simulink model "SVM_CG"  (R2024a)
settings: Solver=FixedStepDiscrete  StartTime=0.0  StopTime=Inf  RelTol=1e-3  EnableMultiTasking=on
undefined symbols (not defined in the file): Down, GPTRIP1SEL, T_period, TZ1, Up, Vdc
libraries: c2802xlib x3, simulink x1
settings Model: ExtModeTrigDuration=8  Creator=kareem  LastModifiedBy=kareem
settings OptimizationCC: DefaultUnderspecifiedDataType=single  EnhancedBackFolding=on  PassReuseOutputArgsAs=Individual arguments  MaxStackSize=1024  OptimizeBlockOrder=speed  DifferentSizesBufferReuse=on  OptimizationCustomize=off  EfficientTunableParamExpr=on
settings DebuggingCC: ParameterTunabilityLossMsg=error
settings HardwareCC: ProdBitPerChar=16  ProdBitPerInt=16  ProdBitPerPointer=32  ProdBitPerSizeT=32  ProdBitPerPtrDiffT=32  ProdLargestAtomicInteger=Integer  ProdLargestAtomicFloat=None  ProdWordSize=16  ProdLongLongMode=on  ProdHWDeviceType=Texas Instruments->C2000  HardwareBoardFeatureSet=SoCBlockset
settings SFSimCC: MATLABDynamicMemAlloc=off
settings RTWCC: Description=Embedded Coder  SystemTargetFile=ert.tlc  HardwareBoard=TI Delfino F28379D LaunchPad  TemplateMakefile=ert_default_tmf  Toolchain=Texas Instruments Code Composer Studio (C2000)  CodeProfilingSaveOptions=MetricsOnly
settings CodeAppCC: ForceParamTrailComments=on  IgnoreCustomStorageClasses=off  OperatorAnnotations=on  SimulinkDataObjDesc=on  SFDataObjDesc=on  InsertBlockDesc=on
settings ERTTargetCC: CodeReplacementLibrary=TI C28x  SupportContinuousTime=on  ExtModeTransport=4  ExtModeStaticAlloc=on  ExtModeAutomaticAllocSize=off  ExtModeStaticAllocSize=10000  ExtModeMexFile=ext_xcp  ExtModeIntrfLevel=Level2 - Open

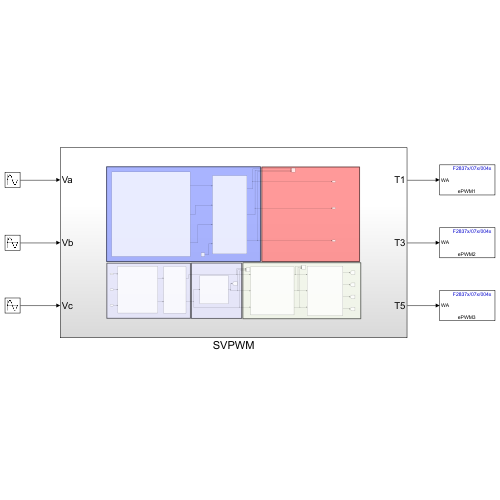
[thumbnail: Simulink's stored preview of the top-level diagram]
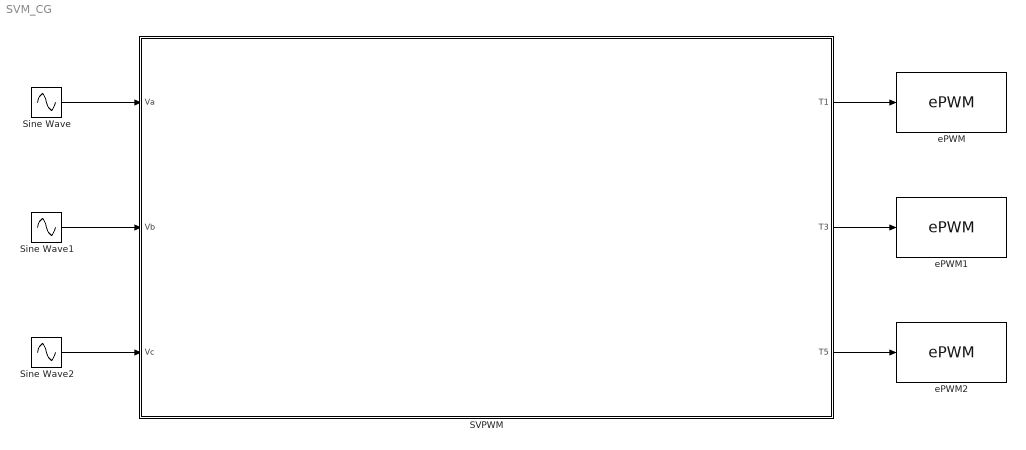
== system SVM_CG ==
  SVPWM : Subsystem
  Sine Wave : Sin  SampleTime=0
  Sine Wave1 : Sin  SampleTime=0
  Sine Wave2 : Sin  SampleTime=0
  ePWM : c2802xlib/ePWM  PwmType=C2000_Type4  useModule=ePWM1  ePWMxLINKTBPRD=Not Linked  periodUnits=Clock cycles  timerSource=Specify via dialog  timerPeriod_clk=10000  timerPeriod_sec=0.0001  tbshadow=Counter equals to zero  countingMode=Up-Down  phaseActiveEnable=Disable  phaseDirection=Count down after sync  phaseActive=0  synchronizationEnable=off  dcaevt1Sync=off  dcbevt1Sync=off  synchronizationOption=Disable  dcbevt1SyncOut=off  dcaevt1SyncOut=off  cmpdSyncOut=off  cmpcSyncOut=off  cmpbSyncOut=off  zeroSyncOut=off  swfSyncOut=off  perSynchronizationOption=Counter equals to period (CTR=PRD)  clockPrescale=1  HSclockPrescale=1  enswap=off  ePWMxAStatus=on  ePWMxAactionLogic1=Do nothing  ePWMxAactionLogic2=Do nothing  ePWMxAactionLogic3=Clear  ePWMxAactionLogic4=Set  ePWMxAactionLogic5=Do nothing  ePWMxAactionLogic6=Do nothing  ePWMxACSFenable=off  ePWMxACSFvalue=Forcing disable  ePWMxASFreload=Zero  ePWMxBStatus=on  ePWMxBactionLogic1=Do nothing  ePWMxBactionLogic2=Do nothing  ePWMxBactionLogic3=Set  ePWMxBactionLogic4=Clear  ePWMxBactionLogic5=Do nothing  ePWMxBactionLogic6=Do nothing  ePWMxBCSFenable=off  ePWMxBCSFvalue=Forcing disable  ePWMxBSFreload=Zero  ePWNxBOutWay=off  ePWMxLINKCMPA=Not Linked  CMPAUnits=Clock cycles  CMPASource=Input port  CMPAValue_per=50  CMPAValue_clk=0  enCMPAshadow=Counter equals to zero (CTR=Zero)  ePWMxLINKCMPB=Not Linked  CMPBUnits=Clock cycles  CMPBSource=Specify via dialog  CMPBValue_per=50  CMPBValue_clk=32000  enCMPBshadow=Counter equals to zero (CTR=Zero)  ePWMxLINKCMPC=Not Linked  CMPCUnits=Clock cycles  CMPCSource=Specify via dialog  CMPCValue_per=50  CMPCValue_clk=32000  enCMPCshadow=Counter equals to zero (CTR=Zero)  ePWMxLINKCMPD=Not Linked  CMPDUnits=Clock cycles  CMPDSource=Specify via dialog  CMPDValue_per=50  CMPDValue_clk=32000  enCMPDshadow=Counter equals to zero (CTR=Zero)  enableDBePWMxA=on  enableDBePWMxB=on  enhalfcycle=off  DBpolarity=Active high complementary (AHC)  DBedgeDelay=Positive  DBSource_ePWMxA=ePWMxA  DBSource_ePWMxB=ePWMxA  DBPeriodUnits=Clock cycles  DBperiodSource=Specify via dialog  REDperiod=400  FEDperiod=400  REDperiod_sec=0  FEDperiod_sec=0  LoadModeDBRED=Immediate without using shadow  LoadModeDBFED=Immediate without using shadow  adcstartModuleA=off  adcrequestEventA=First event  adcstartEventA=Digital Compare Module A Event 1 start of conversion (DCAEVT1.soc)  adcstartEventA_type2=Counter equals to zero (CTR=Zero)  adcstartModuleB=off  adcrequestEventB=First event  adcstartEventB=Counter equals to zero (CTR=Zero)  adcstartEventB_type2=Counter equals to zero (CTR=Zero)  intEn=off  intPrd=First event  intSel=Counter equals to zero (CTR=Zero)  intSel_type2=Counter equals to zero (CTR=Zero)  hrpe=off  enHRPWM=off  HRPWM_LoadMode=Counter equals to period (CTR=PRD)  HRPWM_CTLMode=Duty or Period control mode  HRPWM_EDGMode=Both edge  hrpeb=off  enHRPWMB=off  HRPWM_LoadModeB=Counter equals to zero (CTR=ZERO)  HRPWM_CTLModeB=Duty or Period control mode  HRPWM_EDGModeB=Both edge  enHRDBRED=off  enHRDBFED=off  enSFO=on  enautoconv=on  chopperEnable=off  chopperFrequency=1  chopperFirstwidth=1  chopperDuty=12.5%  tripZonesource=Specify via dialog  tzselOSHT1=off  tzselOSHT2=off  tzselOSHT3=off  tzselOSHT4=off  tzselOSHT5=off  tzselOSHT6=off  tzselOSHDCAEV1=off  tzselOSHDCBEV1=off  tzselCBC1=off  tzselCBC2=off  tzselCBC3=off  tzselCBC4=off  tzselCBC5=off  tzselCBC6=off  tzselCBCDCAEV2=off  tzselCBCDCBEV2=off  enTzOstIntr=off  enTzCbcIntr=off  enTzDCAEVT1Intr=off  enTzDCAEVT2Intr=off  enTzDCBEVT1Intr=off  enTzDCBEVT2Intr=off  tzclrCBCLatch=Counter equals to zero (CTR=Zero)  ePWMxAforced=No action  ePWMxBforced=No action  DCAEVT1forced=No action  DCBEVT1forced=No action  DCAEVT2forced=No action  DCBEVT2forced=No action  dcah=Trip Zone 1 input (TZ1)  dcal=Trip Zone 2 input (TZ2)  dcbh=Trip Zone 1 input (TZ1)  dcbl=Trip Zone 2 input (TZ2)  dcah_type2=GPTRIP1SEL/(TZ1)  dcal_type2=GPTRIP1SEL/(TZ1)  dcbh_type2=GPTRIP1SEL/(TZ1)  dcbl_type2=GPTRIP1SEL/(TZ1)  gendcaevt1=Event disabled  gendcaevt2=Event disabled  gendcbevt1=Event disabled  gendcbevt2=Event disabled  dcaevt1src=DCAEVT1 with sync  dcaevt2src=DCAEVT2 with sync  dcbevt1src=DCBEVT1 with sync  dcbevt2src=DCBEVT2 with sync  pulsesel=Counter equals to zero (CTR=Zero)  blankinv=off  blankoffset=0  blankwidth=0  evsrcsel=Filtered version of DCAEVT1 (DCAEVT1FILT)  encape=off
      settings: LibrarySourceBlock=c2837xDlib/ePWM
  ePWM1 : c2802xlib/ePWM  PwmType=C2000_Type4  useModule=ePWM2  ePWMxLINKTBPRD=Not Linked  periodUnits=Clock cycles  timerSource=Specify via dialog  timerPeriod_clk=10000  timerPeriod_sec=0.0001  tbshadow=Counter equals to zero  countingMode=Up-Down  phaseActiveEnable=Disable  phaseDirection=Count down after sync  phaseActive=0  synchronizationEnable=off  dcaevt1Sync=off  dcbevt1Sync=off  synchronizationOption=Disable  dcbevt1SyncOut=off  dcaevt1SyncOut=off  cmpdSyncOut=off  cmpcSyncOut=off  cmpbSyncOut=off  zeroSyncOut=off  swfSyncOut=off  perSynchronizationOption=Counter equals to period (CTR=PRD)  clockPrescale=1  HSclockPrescale=1  enswap=off  ePWMxAStatus=on  ePWMxAactionLogic1=Do nothing  ePWMxAactionLogic2=Do nothing  ePWMxAactionLogic3=Clear  ePWMxAactionLogic4=Set  ePWMxAactionLogic5=Do nothing  ePWMxAactionLogic6=Do nothing  ePWMxACSFenable=off  ePWMxACSFvalue=Forcing disable  ePWMxASFreload=Zero  ePWMxBStatus=on  ePWMxBactionLogic1=Do nothing  ePWMxBactionLogic2=Do nothing  ePWMxBactionLogic3=Set  ePWMxBactionLogic4=Clear  ePWMxBactionLogic5=Do nothing  ePWMxBactionLogic6=Do nothing  ePWMxBCSFenable=off  ePWMxBCSFvalue=Forcing disable  ePWMxBSFreload=Zero  ePWNxBOutWay=off  ePWMxLINKCMPA=Not Linked  CMPAUnits=Clock cycles  CMPASource=Input port  CMPAValue_per=50  CMPAValue_clk=0  enCMPAshadow=Counter equals to zero (CTR=Zero)  ePWMxLINKCMPB=Not Linked  CMPBUnits=Clock cycles  CMPBSource=Specify via dialog  CMPBValue_per=50  CMPBValue_clk=32000  enCMPBshadow=Counter equals to zero (CTR=Zero)  ePWMxLINKCMPC=Not Linked  CMPCUnits=Clock cycles  CMPCSource=Specify via dialog  CMPCValue_per=50  CMPCValue_clk=32000  enCMPCshadow=Counter equals to zero (CTR=Zero)  ePWMxLINKCMPD=Not Linked  CMPDUnits=Clock cycles  CMPDSource=Specify via dialog  CMPDValue_per=50  CMPDValue_clk=32000  enCMPDshadow=Counter equals to zero (CTR=Zero)  enableDBePWMxA=on  enableDBePWMxB=on  enhalfcycle=off  DBpolarity=Active high complementary (AHC)  DBedgeDelay=Positive  DBSource_ePWMxA=ePWMxA  DBSource_ePWMxB=ePWMxA  DBPeriodUnits=Clock cycles  DBperiodSource=Specify via dialog  REDperiod=400  FEDperiod=400  REDperiod_sec=0  FEDperiod_sec=0  LoadModeDBRED=Immediate without using shadow  LoadModeDBFED=Immediate without using shadow  adcstartModuleA=off  adcrequestEventA=First event  adcstartEventA=Digital Compare Module A Event 1 start of conversion (DCAEVT1.soc)  adcstartEventA_type2=Counter equals to zero (CTR=Zero)  adcstartModuleB=off  adcrequestEventB=First event  adcstartEventB=Counter equals to zero (CTR=Zero)  adcstartEventB_type2=Counter equals to zero (CTR=Zero)  intEn=off  intPrd=First event  intSel=Counter equals to zero (CTR=Zero)  intSel_type2=Counter equals to zero (CTR=Zero)  hrpe=off  enHRPWM=off  HRPWM_LoadMode=Counter equals to period (CTR=PRD)  HRPWM_CTLMode=Duty or Period control mode  HRPWM_EDGMode=Both edge  hrpeb=off  enHRPWMB=off  HRPWM_LoadModeB=Counter equals to zero (CTR=ZERO)  HRPWM_CTLModeB=Duty or Period control mode  HRPWM_EDGModeB=Both edge  enHRDBRED=off  enHRDBFED=off  enSFO=on  enautoconv=on  chopperEnable=off  chopperFrequency=1  chopperFirstwidth=1  chopperDuty=12.5%  tripZonesource=Specify via dialog  tzselOSHT1=off  tzselOSHT2=off  tzselOSHT3=off  tzselOSHT4=off  tzselOSHT5=off  tzselOSHT6=off  tzselOSHDCAEV1=off  tzselOSHDCBEV1=off  tzselCBC1=off  tzselCBC2=off  tzselCBC3=off  tzselCBC4=off  tzselCBC5=off  tzselCBC6=off  tzselCBCDCAEV2=off  tzselCBCDCBEV2=off  enTzOstIntr=off  enTzCbcIntr=off  enTzDCAEVT1Intr=off  enTzDCAEVT2Intr=off  enTzDCBEVT1Intr=off  enTzDCBEVT2Intr=off  tzclrCBCLatch=Counter equals to zero (CTR=Zero)  ePWMxAforced=No action  ePWMxBforced=No action  DCAEVT1forced=No action  DCBEVT1forced=No action  DCAEVT2forced=No action  DCBEVT2forced=No action  dcah=Trip Zone 1 input (TZ1)  dcal=Trip Zone 2 input (TZ2)  dcbh=Trip Zone 1 input (TZ1)  dcbl=Trip Zone 2 input (TZ2)  dcah_type2=GPTRIP1SEL/(TZ1)  dcal_type2=GPTRIP1SEL/(TZ1)  dcbh_type2=GPTRIP1SEL/(TZ1)  dcbl_type2=GPTRIP1SEL/(TZ1)  gendcaevt1=Event disabled  gendcaevt2=Event disabled  gendcbevt1=Event disabled  gendcbevt2=Event disabled  dcaevt1src=DCAEVT1 with sync  dcaevt2src=DCAEVT2 with sync  dcbevt1src=DCBEVT1 with sync  dcbevt2src=DCBEVT2 with sync  pulsesel=Counter equals to zero (CTR=Zero)  blankinv=off  blankoffset=0  blankwidth=0  evsrcsel=Filtered version of DCAEVT1 (DCAEVT1FILT)  encape=off
      settings: LibrarySourceBlock=c2837xDlib/ePWM
  ePWM2 : c2802xlib/ePWM  PwmType=C2000_Type4  useModule=ePWM3  ePWMxLINKTBPRD=Not Linked  periodUnits=Clock cycles  timerSource=Specify via dialog  timerPeriod_clk=10000  timerPeriod_sec=0.0001  tbshadow=Counter equals to zero  countingMode=Up-Down  phaseActiveEnable=Disable  phaseDirection=Count down after sync  phaseActive=0  synchronizationEnable=off  dcaevt1Sync=off  dcbevt1Sync=off  synchronizationOption=Disable  dcbevt1SyncOut=off  dcaevt1SyncOut=off  cmpdSyncOut=off  cmpcSyncOut=off  cmpbSyncOut=off  zeroSyncOut=off  swfSyncOut=off  perSynchronizationOption=Counter equals to period (CTR=PRD)  clockPrescale=1  HSclockPrescale=1  enswap=off  ePWMxAStatus=on  ePWMxAactionLogic1=Do nothing  ePWMxAactionLogic2=Do nothing  ePWMxAactionLogic3=Clear  ePWMxAactionLogic4=Set  ePWMxAactionLogic5=Do nothing  ePWMxAactionLogic6=Do nothing  ePWMxACSFenable=off  ePWMxACSFvalue=Forcing disable  ePWMxASFreload=Zero  ePWMxBStatus=on  ePWMxBactionLogic1=Do nothing  ePWMxBactionLogic2=Do nothing  ePWMxBactionLogic3=Set  ePWMxBactionLogic4=Clear  ePWMxBactionLogic5=Do nothing  ePWMxBactionLogic6=Do nothing  ePWMxBCSFenable=off  ePWMxBCSFvalue=Forcing disable  ePWMxBSFreload=Zero  ePWNxBOutWay=off  ePWMxLINKCMPA=Not Linked  CMPAUnits=Clock cycles  CMPASource=Input port  CMPAValue_per=50  CMPAValue_clk=0  enCMPAshadow=Counter equals to zero (CTR=Zero)  ePWMxLINKCMPB=Not Linked  CMPBUnits=Clock cycles  CMPBSource=Specify via dialog  CMPBValue_per=50  CMPBValue_clk=32000  enCMPBshadow=Counter equals to zero (CTR=Zero)  ePWMxLINKCMPC=Not Linked  CMPCUnits=Clock cycles  CMPCSource=Specify via dialog  CMPCValue_per=50  CMPCValue_clk=32000  enCMPCshadow=Counter equals to zero (CTR=Zero)  ePWMxLINKCMPD=Not Linked  CMPDUnits=Clock cycles  CMPDSource=Specify via dialog  CMPDValue_per=50  CMPDValue_clk=32000  enCMPDshadow=Counter equals to zero (CTR=Zero)  enableDBePWMxA=on  enableDBePWMxB=on  enhalfcycle=off  DBpolarity=Active high complementary (AHC)  DBedgeDelay=Positive  DBSource_ePWMxA=ePWMxA  DBSource_ePWMxB=ePWMxA  DBPeriodUnits=Clock cycles  DBperiodSource=Specify via dialog  REDperiod=400  FEDperiod=400  REDperiod_sec=0  FEDperiod_sec=0  LoadModeDBRED=Immediate without using shadow  LoadModeDBFED=Immediate without using shadow  adcstartModuleA=off  adcrequestEventA=First event  adcstartEventA=Digital Compare Module A Event 1 start of conversion (DCAEVT1.soc)  adcstartEventA_type2=Counter equals to zero (CTR=Zero)  adcstartModuleB=off  adcrequestEventB=First event  adcstartEventB=Counter equals to zero (CTR=Zero)  adcstartEventB_type2=Counter equals to zero (CTR=Zero)  intEn=off  intPrd=First event  intSel=Counter equals to zero (CTR=Zero)  intSel_type2=Counter equals to zero (CTR=Zero)  hrpe=off  enHRPWM=off  HRPWM_LoadMode=Counter equals to period (CTR=PRD)  HRPWM_CTLMode=Duty or Period control mode  HRPWM_EDGMode=Both edge  hrpeb=off  enHRPWMB=off  HRPWM_LoadModeB=Counter equals to zero (CTR=ZERO)  HRPWM_CTLModeB=Duty or Period control mode  HRPWM_EDGModeB=Both edge  enHRDBRED=off  enHRDBFED=off  enSFO=on  enautoconv=on  chopperEnable=off  chopperFrequency=1  chopperFirstwidth=1  chopperDuty=12.5%  tripZonesource=Specify via dialog  tzselOSHT1=off  tzselOSHT2=off  tzselOSHT3=off  tzselOSHT4=off  tzselOSHT5=off  tzselOSHT6=off  tzselOSHDCAEV1=off  tzselOSHDCBEV1=off  tzselCBC1=off  tzselCBC2=off  tzselCBC3=off  tzselCBC4=off  tzselCBC5=off  tzselCBC6=off  tzselCBCDCAEV2=off  tzselCBCDCBEV2=off  enTzOstIntr=off  enTzCbcIntr=off  enTzDCAEVT1Intr=off  enTzDCAEVT2Intr=off  enTzDCBEVT1Intr=off  enTzDCBEVT2Intr=off  tzclrCBCLatch=Counter equals to zero (CTR=Zero)  ePWMxAforced=No action  ePWMxBforced=No action  DCAEVT1forced=No action  DCBEVT1forced=No action  DCAEVT2forced=No action  DCBEVT2forced=No action  dcah=Trip Zone 1 input (TZ1)  dcal=Trip Zone 2 input (TZ2)  dcbh=Trip Zone 1 input (TZ1)  dcbl=Trip Zone 2 input (TZ2)  dcah_type2=GPTRIP1SEL/(TZ1)  dcal_type2=GPTRIP1SEL/(TZ1)  dcbh_type2=GPTRIP1SEL/(TZ1)  dcbl_type2=GPTRIP1SEL/(TZ1)  gendcaevt1=Event disabled  gendcaevt2=Event disabled  gendcbevt1=Event disabled  gendcbevt2=Event disabled  dcaevt1src=DCAEVT1 with sync  dcaevt2src=DCAEVT2 with sync  dcbevt1src=DCBEVT1 with sync  dcbevt2src=DCBEVT2 with sync  pulsesel=Counter equals to zero (CTR=Zero)  blankinv=off  blankoffset=0  blankwidth=0  evsrcsel=Filtered version of DCAEVT1 (DCAEVT1FILT)  encape=off
      settings: LibrarySourceBlock=c2837xDlib/ePWM
  wires:
  Sine Wave2/1 -> SVPWM/3(Vc)
  Sine Wave1/1 -> SVPWM/2(Vb)
  Sine Wave/1 -> SVPWM/1(Va)
  SVPWM/3(T5) -> ePWM2/1
  SVPWM/2(T3) -> ePWM1/1
  SVPWM/1(T1) -> ePWM/1

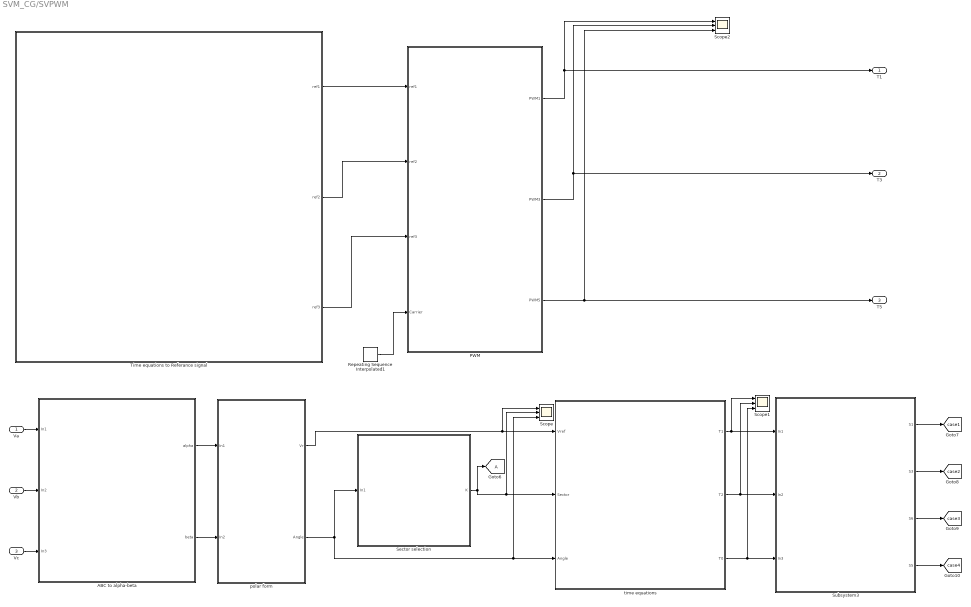
== system SVM_CG/SVPWM ==
  Va : Inport
  Vb : Inport  Port=2
  Vc : Inport  Port=3
  ABC to alpha-beta : Subsystem
  Goto6 : Goto  TagVisibility=global
  PWM : Subsystem
  Repeating Sequence Interpolated1 : simulink/Sources/Repeating Sequence Interpolated  OutValues="[ 0 1/15000  1e-6  ]"  TimeValues=[ 0 1/40000 1/20001]  LookUpMeth=Interpolation-Use End Values  tsamp=1e-6  OutMin=[]  OutMax=[]  OutDataTypeStr=double  OutputDataTypeScalingMode=double  OutDataType=fixdt(0,8)  OutScaling=2^-10
  Scope : Scope  NumInputPorts=3
  Scope1 : Scope  NumInputPorts=3
  Scope2 : Scope  NumInputPorts=3
  Sector selection : Subsystem
  Subsystem3 : Subsystem
  Time equations to Referance signal : Subsystem
  polar form : Subsystem
  time equations : Subsystem
  T1 : Outport
  T3 : Outport  Port=2
  T5 : Outport  Port=3
  tag scope: case1=global, case2=global, case3=global, case4=global
  wires:
  Vb/1 -> ABC to alpha-beta/2(In2)
  time equations/1(T1) -> Scope1/1, Subsystem3/1(In1)
  Va/1 -> ABC to alpha-beta/1(In1)
  Time equations to Referance signal/1(ref1) -> PWM/1(ref1)
  Time equations to Referance signal/2("ref2 ") -> PWM/2(ref2)
  Time equations to Referance signal/3(ref3) -> PWM/3(ref3)
  Vc/1 -> ABC to alpha-beta/3(In3)
  ABC to alpha-beta/1(alpha) -> polar form/1(In1)
  ABC to alpha-beta/2(beta) -> polar form/2(In2)
  PWM/1(PWM1) -> T1/1, Scope2/1
  PWM/2(PWM3) -> T3/1, Scope2/2
  PWM/3(PWM5) -> T5/1, Scope2/3
  polar form/2(Angle) -> Sector selection/1(In1), time equations/3(Angle), Scope/3
  polar form/1(Vr) -> Scope/1, time equations/1(Vref)
  Sector selection/1(K) -> Scope/2, time equations/2(Sector), Goto6/1
  Subsystem3/2(S3) -> [case2]
  Subsystem3/1(S1) -> [case1]
  time equations/3(T0) -> Subsystem3/3(In3), Scope1/3
  time equations/2(T2) -> Scope1/2, Subsystem3/2(In2)
  Subsystem3/4(S5) -> [case4]
  Subsystem3/3(S6) -> [case3]
  Repeating Sequence Interpolated1/1 -> PWM/4(Carrier)

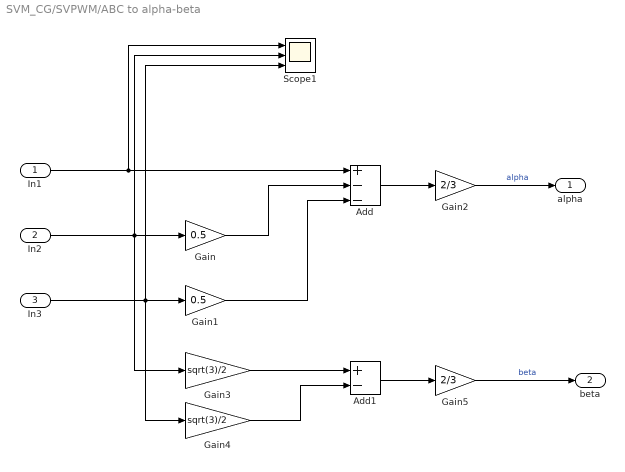
== system SVM_CG/SVPWM/ABC to alpha-beta ==
  In1 : Inport
  In2 : Inport  Port=2
  In3 : Inport  Port=3
  Add : Sum  Inputs=+--
  Add1 : Sum  Inputs=+-
  Gain : Gain  Gain=0.5
  Gain1 : Gain  Gain=0.5
  Gain2 : Gain  Gain=2/3
  Gain3 : Gain  Gain=sqrt(3)/2
  Gain4 : Gain  Gain=sqrt(3)/2
  Gain5 : Gain  Gain=2/3
  Scope1 : Scope  NumInputPorts=3
  alpha : Outport
  beta : Outport  Port=2
  wires:
  Gain3/1 -> Add1/1
  In2/1 -> Gain3/1, Scope1/2, Gain/1
  Gain4/1 -> Add1/2
  Add1/1 -> Gain5/1
  Gain1/1 -> Add/3
  In3/1 -> Scope1/3, Gain4/1, Gain1/1
  Gain/1 -> Add/2
  In1/1 -> Add/1, Scope1/1
  Add/1 -> Gain2/1
  Gain2/1 -> alpha/1  "alpha"
  Gain5/1 -> beta/1  "beta"

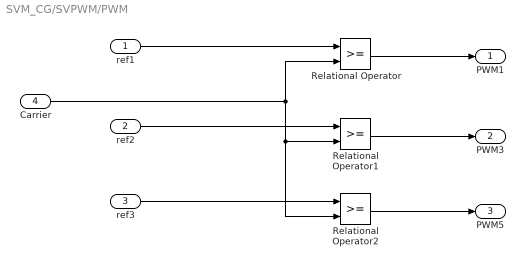
== system SVM_CG/SVPWM/PWM ==
  ref1 : Inport
  ref2 : Inport  Port=2
  ref3 : Inport  Port=3
  Carrier : Inport  Port=4
  Relational Operator : RelationalOperator  OutDataTypeStr=boolean  RndMeth=Simplest  InputSameDT=off
  Relational Operator1 : RelationalOperator  OutDataTypeStr=boolean  RndMeth=Simplest  InputSameDT=off
  Relational Operator2 : RelationalOperator  OutDataTypeStr=boolean  RndMeth=Simplest  InputSameDT=off
  PWM1 : Outport
  PWM3 : Outport  Port=2
  PWM5 : Outport  Port=3
  wires:
  ref1/1 -> Relational Operator/1
  ref2/1 -> Relational Operator1/1
  ref3/1 -> Relational Operator2/1
  Carrier/1 -> Relational Operator/2, Relational Operator2/2, Relational Operator1/2
  Relational Operator/1 -> PWM1/1
  Relational Operator1/1 -> PWM3/1
  Relational Operator2/1 -> PWM5/1

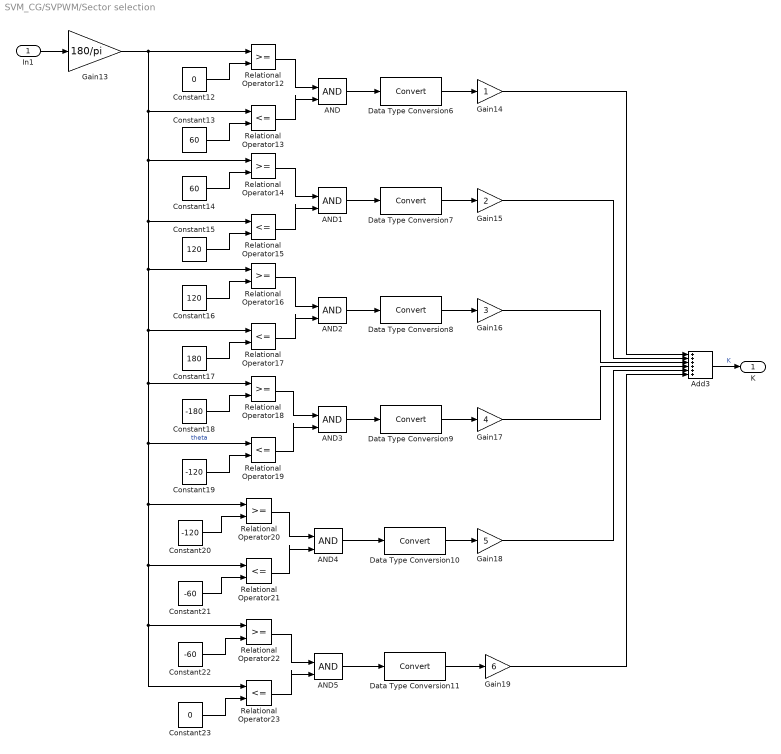
== system SVM_CG/SVPWM/Sector selection ==
  In1 : Inport
  AND{,1..5} (6 alike) : Logic  IconShape=distinctive  AllPortsSameDT=off  OutDataTypeStr=boolean
  Add3 : Sum  Inputs=++++++
  Constant12 : Constant  Value=0
  Constant13 : Constant  Value=60
  Constant14 : Constant  Value=60
  Constant15 : Constant  Value=120
  Constant16 : Constant  Value=120
  Constant17 : Constant  Value=180
  Constant18 : Constant  Value=-180
  Constant19 : Constant  Value=-120
  Constant20 : Constant  Value=-120
  Constant21 : Constant  Value=-60
  Constant22 : Constant  Value=-60
  Constant23 : Constant  Value=0
  Data Type Conversion{6..11} (6 alike) : DataTypeConversion  SaturateOnIntegerOverflow=off  RndMeth=Floor
  Gain13 : Gain  Gain=180/pi
  Gain14 : Gain
  Gain15 : Gain  Gain=2
  Gain16 : Gain  Gain=3
  Gain17 : Gain  Gain=4
  Gain18 : Gain  Gain=5
  Gain19 : Gain  Gain=6
  Relational Operator{12,14,16,18,20,22} (6 alike) : RelationalOperator  OutDataTypeStr=boolean  RndMeth=Simplest  InputSameDT=off
  Relational Operator{13,15,17,19,21,23} (6 alike) : RelationalOperator  Operator=<=  OutDataTypeStr=boolean  RndMeth=Simplest  InputSameDT=off
  K : Outport
  wires:
  AND2/1 -> Data Type Conversion8/1
  Relational Operator14/1 -> AND1/1
  Relational Operator12/1 -> AND/1
  Data Type Conversion10/1 -> Gain18/1
  Data Type Conversion8/1 -> Gain16/1
  Relational Operator19/1 -> AND3/2
  Gain13/1 -> Relational Operator14/1, Relational Operator18/1, Relational Operator19/1, Relational Operator20/1, Relational Operator22/1, Relational Operator23/1, Relational Operator21/1, Relational Operator17/1, Relational Operator16/1, Relational Operator15/1, Relational Operator13/1, Relational Operator12/1  "theta"
  Data Type Conversion6/1 -> Gain14/1
  Constant21/1 -> Relational Operator21/2
  Constant19/1 -> Relational Operator19/2
  Gain19/1 -> Add3/6
  Constant18/1 -> Relational Operator18/2
  AND4/1 -> Data Type Conversion10/1
  Constant22/1 -> Relational Operator22/2
  Relational Operator22/1 -> AND5/1
  Relational Operator18/1 -> AND3/1
  Gain15/1 -> Add3/2
  Relational Operator23/1 -> AND5/2
  Data Type Conversion11/1 -> Gain19/1
  Constant16/1 -> Relational Operator16/2
  Data Type Conversion7/1 -> Gain15/1
  Constant23/1 -> Relational Operator23/2
  Relational Operator20/1 -> AND4/1
  Gain18/1 -> Add3/5
  Gain14/1 -> Add3/1
  AND1/1 -> Data Type Conversion7/1
  Constant14/1 -> Relational Operator14/2
  Relational Operator16/1 -> AND2/1
  Relational Operator17/1 -> AND2/2
  Gain17/1 -> Add3/4
  Constant12/1 -> Relational Operator12/2
  Gain16/1 -> Add3/3
  Relational Operator13/1 -> AND/2
  Relational Operator15/1 -> AND1/2
  Data Type Conversion9/1 -> Gain17/1
  AND/1 -> Data Type Conversion6/1
  Constant13/1 -> Relational Operator13/2
  Relational Operator21/1 -> AND4/2
  AND3/1 -> Data Type Conversion9/1
  Constant20/1 -> Relational Operator20/2
  Constant17/1 -> Relational Operator17/2
  AND5/1 -> Data Type Conversion11/1
  Constant15/1 -> Relational Operator15/2
  Add3/1 -> K/1  "K"
  In1/1 -> Gain13/1

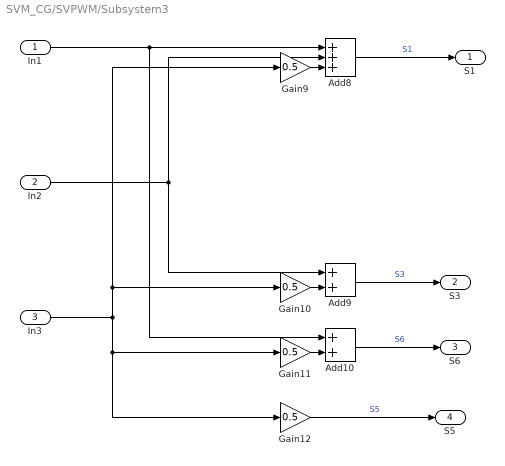
== system SVM_CG/SVPWM/Subsystem3 ==
  In1 : Inport
  In2 : Inport  Port=2
  In3 : Inport  Port=3
  Add10 : Sum
  Add8 : Sum  Inputs=+++
  Add9 : Sum
  Gain{9..12} (4 alike) : Gain  Gain=0.5
  S1 : Outport
  S3 : Outport  Port=2
  S6 : Outport  Port=3
  S5 : Outport  Port=4
  wires:
  In3/1 -> Gain9/1, Gain10/1, Gain12/1, Gain11/1
  Gain11/1 -> Add10/2
  Gain9/1 -> Add8/3
  Gain10/1 -> Add9/2
  Add8/1 -> S1/1  "S1"
  In2/1 -> Add9/1, Add8/2
  In1/1 -> Add10/1, Add8/1
  Add9/1 -> S3/1  "S3"
  Gain12/1 -> S5/1  "S5"
  Add10/1 -> S6/1  "S6"

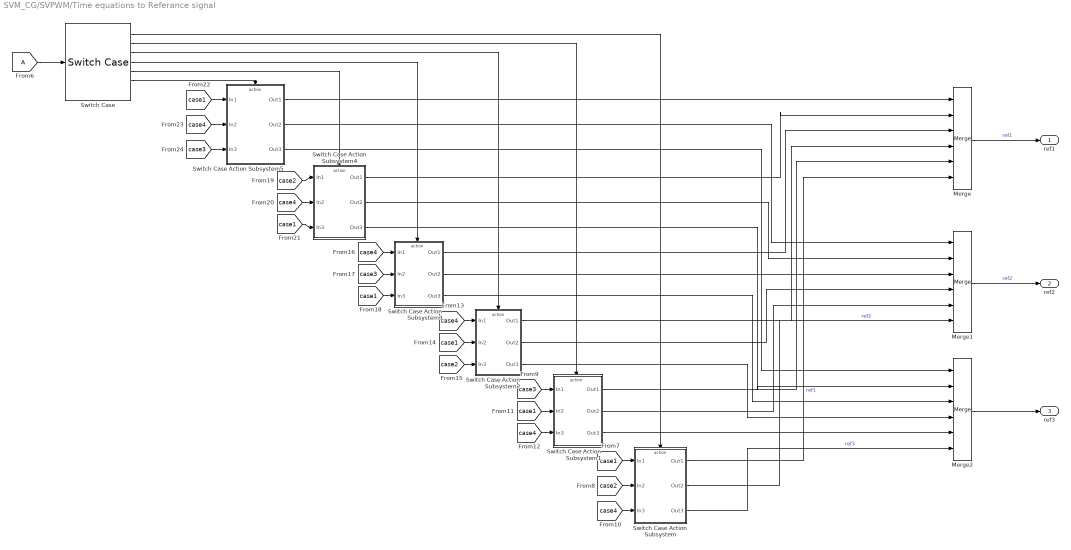
== system SVM_CG/SVPWM/Time equations to Referance signal ==
  From6 : From  TagVisibility=global
  Merge : Merge  Inputs=6
  Merge1 : Merge  Inputs=6
  Merge2 : Merge  Inputs=6
  Switch Case : SwitchCase  CaseConditions={1 2 3 4 5 6}
  Switch Case Action Subsystem : Subsystem  TreatAsAtomicUnit=on
  Switch Case Action Subsystem1 : Subsystem  TreatAsAtomicUnit=on
  Switch Case Action Subsystem2 : Subsystem  TreatAsAtomicUnit=on
  Switch Case Action Subsystem3 : Subsystem  TreatAsAtomicUnit=on
  Switch Case Action Subsystem4 : Subsystem  TreatAsAtomicUnit=on
  Switch Case Action Subsystem5 : Subsystem  TreatAsAtomicUnit=on
  ref1 : Outport
  "ref2 " : Outport  Port=2
  ref3 : Outport  Port=3
  wires:
  [case3] -> Switch Case Action Subsystem5/3(In3)
  Switch Case Action Subsystem4/1(Out1) -> Merge/2
  [case1] -> Switch Case Action Subsystem2/2(In2)
  Switch Case Action Subsystem3/2(Out2) -> Merge1/3
  [case4] -> Switch Case Action Subsystem3/1(In1)
  Switch Case/4 -> Switch Case Action Subsystem3/Action
  [case2] -> Switch Case Action Subsystem4/1(In1)
  Switch Case/6 -> Switch Case Action Subsystem5/Action
  [case4] -> Switch Case Action Subsystem1/3(In3)
  [case1] -> Switch Case Action Subsystem5/1(In1)
  [case3] -> Switch Case Action Subsystem1/1(In1)
  Merge/1 -> ref1/1  "ref1"
  Switch Case Action Subsystem5/1(Out1) -> Merge/1
  Switch Case/5 -> Switch Case Action Subsystem4/Action
  Switch Case Action Subsystem4/3(Out3) -> Merge2/2
  [case1] -> Switch Case Action Subsystem/1(In1)
  Switch Case Action Subsystem2/3(Out3) -> Merge2/4
  Switch Case Action Subsystem4/2(Out2) -> Merge1/2
  Switch Case/3 -> Switch Case Action Subsystem2/Action
  Switch Case Action Subsystem/2(Out2) -> Merge1/6  "ref2"
  Switch Case Action Subsystem3/3(Out3) -> Merge2/3
  Switch Case Action Subsystem5/2(Out2) -> Merge1/1
  [case3] -> Switch Case Action Subsystem3/2(In2)
  Switch Case/2 -> Switch Case Action Subsystem1/Action
  Switch Case Action Subsystem2/1(Out1) -> Merge/4
  Switch Case Action Subsystem2/2(Out2) -> Merge1/4
  [case1] -> Switch Case Action Subsystem4/3(In3)
  [case4] -> Switch Case Action Subsystem5/2(In2)
  Switch Case/1 -> Switch Case Action Subsystem/Action
  Switch Case Action Subsystem5/3(Out3) -> Merge2/1
  [case4] -> Switch Case Action Subsystem2/1(In1)
  Switch Case Action Subsystem3/1(Out1) -> Merge/3
  [case4] -> Switch Case Action Subsystem/3(In3)
  Merge2/1 -> ref3/1
  From6/1 -> Switch Case/1
  [case4] -> Switch Case Action Subsystem4/2(In2)
  [case2] -> Switch Case Action Subsystem/2(In2)
  [case2] -> Switch Case Action Subsystem2/3(In3)
  [case1] -> Switch Case Action Subsystem3/3(In3)
  Switch Case Action Subsystem1/2(Out2) -> Merge1/5
  Switch Case Action Subsystem/1(Out1) -> Merge/6  "ref1"
  Switch Case Action Subsystem1/1(Out1) -> Merge/5
  Switch Case Action Subsystem/3(Out3) -> Merge2/6  "ref3"
  Switch Case Action Subsystem1/3(Out3) -> Merge2/5
  [case1] -> Switch Case Action Subsystem1/2(In2)
  Merge1/1 -> "ref2 "/1  "ref2"

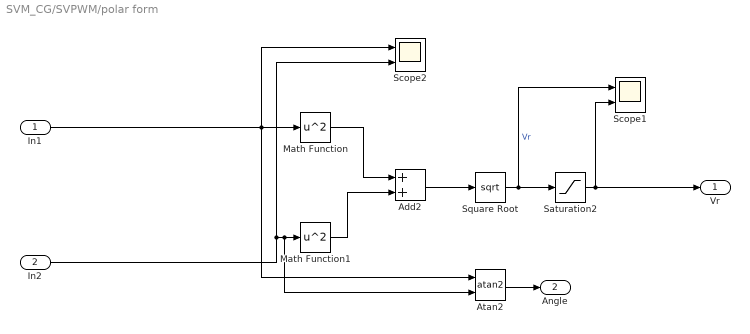
== system SVM_CG/SVPWM/polar form ==
  In1 : Inport
  In2 : Inport  Port=2
  Add2 : Sum
  Atan2 : Trigonometry  Operator=atan2
  Math Function : Math  Operator=square  SignedPower=on
  Math Function1 : Math  Operator=square  SignedPower=on
  Saturation2 : Saturate  UpperLimit=0.95 * Vdc /sqrt(3)  LowerLimit=0
  Scope1 : Scope  NumInputPorts=2
  Scope2 : Scope  NumInputPorts=2
  Square Root : Sqrt
  Vr : Outport
  Angle : Outport  Port=2
  wires:
  In2/1 -> Scope2/2, Atan2/2, Math Function1/1
  In1/1 -> Scope2/1, Atan2/1, Math Function/1
  Math Function1/1 -> Add2/2
  Add2/1 -> Square Root/1
  Math Function/1 -> Add2/1
  Atan2/1 -> Angle/1
  Square Root/1 -> Saturation2/1, Scope1/1  "Vr"
  Saturation2/1 -> Vr/1, Scope1/2

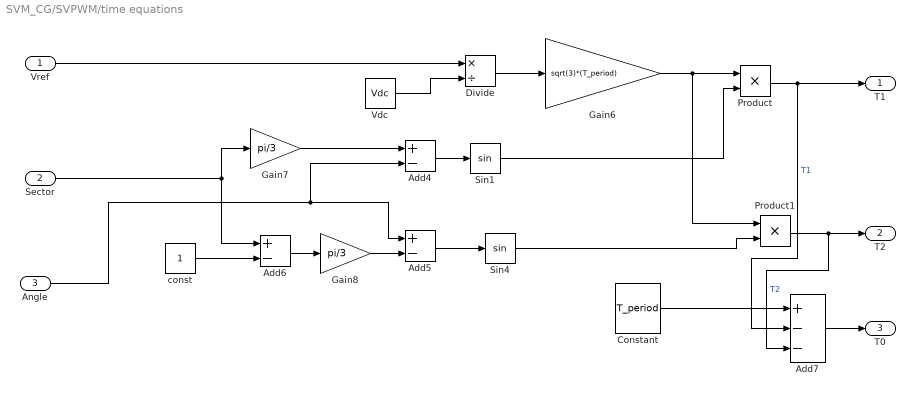
== system SVM_CG/SVPWM/time equations ==
  Vref : Inport
  Sector : Inport  Port=2
  Angle : Inport  Port=3
  Add4 : Sum  Inputs=+-
  Add5 : Sum  Inputs=+-
  Add6 : Sum  Inputs=+-
  Add7 : Sum  Inputs=+--
  Constant : Constant  Value=T_period
  Divide : Product  Inputs=*/
  Gain6 : Gain  Gain=sqrt(3)*(T_period)
  Gain7 : Gain  Gain=pi/3
  Gain8 : Gain  Gain=pi/3
  Product : Product
  Product1 : Product
  Sin1 : Trigonometry
  Sin4 : Trigonometry
  Vdc : Constant  Value=Vdc
  const : Constant
  T1 : Outport
  T2 : Outport  Port=2
  T0 : Outport  Port=3
  wires:
  Vdc/1 -> Divide/2
  Gain6/1 -> Product1/1, Product/1
  Divide/1 -> Gain6/1
  Add6/1 -> Gain8/1
  Constant/1 -> Add7/1
  Gain7/1 -> Add4/1
  Add5/1 -> Sin4/1
  Sin4/1 -> Product1/2
  Sin1/1 -> Product/2
  Gain8/1 -> Add5/2
  Angle/1 -> Add5/1, Add4/2
  const/1 -> Add6/2
  Product1/1 -> T2/1, Add7/3  "T2"
  Sector/1 -> Gain7/1, Add6/1
  Add4/1 -> Sin1/1
  Vref/1 -> Divide/1
  Product/1 -> Add7/2, T1/1  "T1"
  Add7/1 -> T0/1

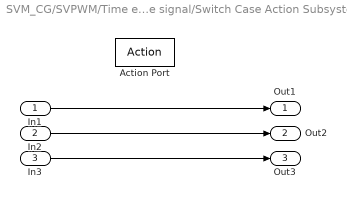
== system SVM_CG/SVPWM/Time equations to Referance signal/Switch Case Action Subsystem ==
  In1 : Inport
  In2 : Inport  Port=2
  In3 : Inport  Port=3
  Action Port : ActionPort  ActionPortLabel=case [ 1 ]:
  Out1 : Outport
  Out2 : Outport  Port=2
  Out3 : Outport  Port=3
  wires:
  In1/1 -> Out1/1
  In2/1 -> Out2/1
  In3/1 -> Out3/1

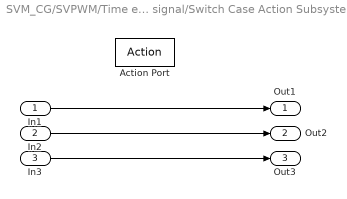
== system SVM_CG/SVPWM/Time equations to Referance signal/Switch Case Action Subsystem1 ==
  In1 : Inport
  In2 : Inport  Port=2
  In3 : Inport  Port=3
  Action Port : ActionPort  ActionPortLabel=case [ 2 ]:
  Out1 : Outport
  Out2 : Outport  Port=2
  Out3 : Outport  Port=3
  wires:
  In1/1 -> Out1/1
  In2/1 -> Out2/1
  In3/1 -> Out3/1

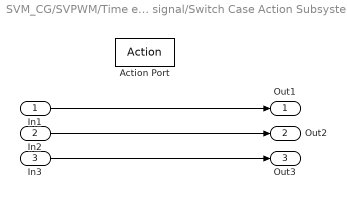
== system SVM_CG/SVPWM/Time equations to Referance signal/Switch Case Action Subsystem2 ==
  In1 : Inport
  In2 : Inport  Port=2
  In3 : Inport  Port=3
  Action Port : ActionPort  ActionPortLabel=case [ 3 ]:
  Out1 : Outport
  Out2 : Outport  Port=2
  Out3 : Outport  Port=3
  wires:
  In1/1 -> Out1/1
  In2/1 -> Out2/1
  In3/1 -> Out3/1

== system SVM_CG/SVPWM/Time equations to Referance signal/Switch Case Action Subsystem3 ==
  In1 : Inport
  In2 : Inport  Port=2
  In3 : Inport  Port=3
  Action Port : ActionPort  ActionPortLabel=case [ 4 ]:
  Out1 : Outport
  Out2 : Outport  Port=2
  Out3 : Outport  Port=3
  wires:
  In1/1 -> Out1/1
  In2/1 -> Out2/1
  In3/1 -> Out3/1

== system SVM_CG/SVPWM/Time equations to Referance signal/Switch Case Action Subsystem4 ==
  In1 : Inport
  In2 : Inport  Port=2
  In3 : Inport  Port=3
  Action Port : ActionPort  ActionPortLabel=case [ 5 ]:
  Out1 : Outport
  Out2 : Outport  Port=2
  Out3 : Outport  Port=3
  wires:
  In1/1 -> Out1/1
  In2/1 -> Out2/1
  In3/1 -> Out3/1

== system SVM_CG/SVPWM/Time equations to Referance signal/Switch Case Action Subsystem5 ==
  In1 : Inport
  In2 : Inport  Port=2
  In3 : Inport  Port=3
  Action Port : ActionPort  ActionPortLabel=case [ 6 ]:
  Out1 : Outport
  Out2 : Outport  Port=2
  Out3 : Outport  Port=3
  wires:
  In1/1 -> Out1/1
  In2/1 -> Out2/1
  In3/1 -> Out3/1
